simulink model "assignment3"  (R2016a)
settings: Solver=VariableStepAuto  StartTime=0.0  StopTime=1000  RelTol=1e-3
values from neighbouring files (symbols this model uses):
  f_ref = 0    [assgt3.m]
  Ki_f = 1/Ti_f    (= 0.215982721382)    [assgt3.m]
  Ki_p = 1/Ti_p    (= 0.289855072464)    [assgt3.m]
  Kp_f = 3.04    [assgt3.m]
  Kp_p = 18    [assgt3.m]
  p_ref = 0    [assgt3.m]
  Ti_f = 4.63    [assgt3.m]
  Ti_p = 3.45    [assgt3.m]
settings Model: Creator=Sondre  LastModifiedBy=Sondre

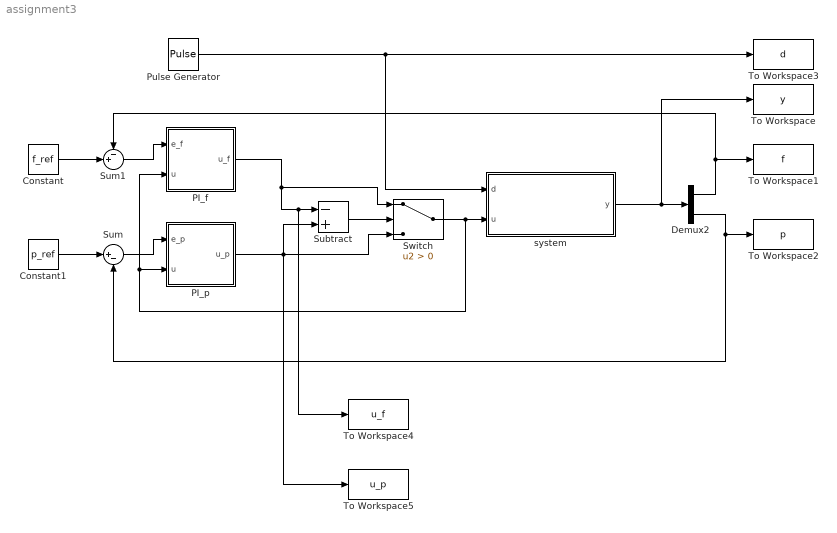
== system assignment3 ==
  Constant : Constant  Value=f_ref
  Constant1 : Constant  Value=p_ref
  Demux2 : Demux  Outputs=2
  PI_f : Subsystem
  PI_p : Subsystem
  Pulse Generator : DiscretePulseGenerator  PulseType=Time based  Period=500  PulseWidth=50
  Subtract : Sum  Inputs=-+
  Sum : Sum  Inputs=|+-
  Sum1 : Sum  Inputs=-+|
  Switch : Switch  Criteria=u2 > Threshold
  To Workspace : ToWorkspace  VariableName=y  SaveFormat=Timeseries  SampleTime=-1
  To Workspace1 : ToWorkspace  VariableName=f  SaveFormat=Timeseries  SampleTime=-1
  To Workspace2 : ToWorkspace  VariableName=p  SaveFormat=Timeseries  SampleTime=-1
  To Workspace3 : ToWorkspace  VariableName=d  SaveFormat=Timeseries  SampleTime=-1
  To Workspace4 : ToWorkspace  VariableName=u_f  SaveFormat=Timeseries  SampleTime=-1
  To Workspace5 : ToWorkspace  VariableName=u_p  SaveFormat=Timeseries  SampleTime=-1
  system : Subsystem
  wires:
  Demux2/2 -> Sum/2, To Workspace2/1
  system/1("y ") -> Demux2/1, To Workspace/1
  Constant1/1 -> Sum/1
  Sum/1 -> PI_p/1("e_p ")
  Sum1/1 -> PI_f/1("e_f ")
  PI_f/1("u_f ") -> Switch/1, To Workspace4/1, Subtract/1
  Pulse Generator/1 -> To Workspace3/1, system/1(d)
  Constant/1 -> Sum1/2
  Demux2/1 -> Sum1/1, To Workspace1/1
  PI_p/1("u_p ") -> To Workspace5/1, Subtract/2, Switch/3
  Subtract/1 -> Switch/2
  Switch/1 -> PI_f/2(u), PI_p/2("u "), system/2("u ")

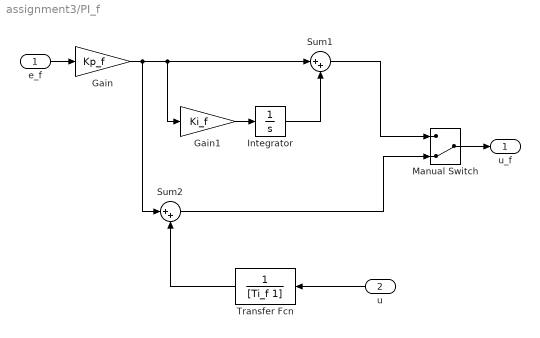
== system assignment3/PI_f ==
  "e_f " : Inport
  u : Inport  Port=2
  Gain : Gain  Gain=Kp_f
  Gain1 : Gain  Gain=Ki_f
  Integrator : Integrator
  Manual Switch : ManualSwitch  CurrentSetting=0
  Sum1 : Sum  Inputs=|++
  Sum2 : Sum  Inputs=|++
  Transfer Fcn : TransferFcn  Denominator=[Ti_f 1]
  "u_f " : Outport
  wires:
  Gain1/1 -> Integrator/1
  Integrator/1 -> Sum1/2
  "e_f "/1 -> Gain/1
  Gain/1 -> Sum2/1, Gain1/1, Sum1/1
  Sum2/1 -> Manual Switch/2
  Transfer Fcn/1 -> Sum2/2
  Manual Switch/1 -> "u_f "/1
  Sum1/1 -> Manual Switch/1
  u/1 -> Transfer Fcn/1

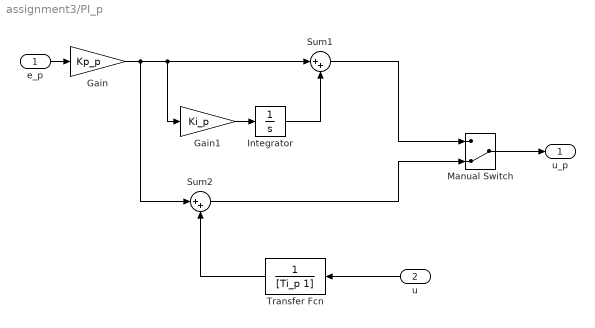
== system assignment3/PI_p ==
  "e_p " : Inport
  "u " : Inport  Port=2
  Gain : Gain  Gain=Kp_p
  Gain1 : Gain  Gain=Ki_p
  Integrator : Integrator
  Manual Switch : ManualSwitch  CurrentSetting=0
  Sum1 : Sum  Inputs=|++
  Sum2 : Sum  Inputs=|++
  Transfer Fcn : TransferFcn  Denominator=[Ti_p 1]
  "u_p " : Outport
  wires:
  Gain1/1 -> Integrator/1
  Integrator/1 -> Sum1/2
  "e_p "/1 -> Gain/1
  Gain/1 -> Sum2/1, Gain1/1, Sum1/1
  Sum2/1 -> Manual Switch/2
  Transfer Fcn/1 -> Sum2/2
  Manual Switch/1 -> "u_p "/1
  Sum1/1 -> Manual Switch/1
  "u "/1 -> Transfer Fcn/1

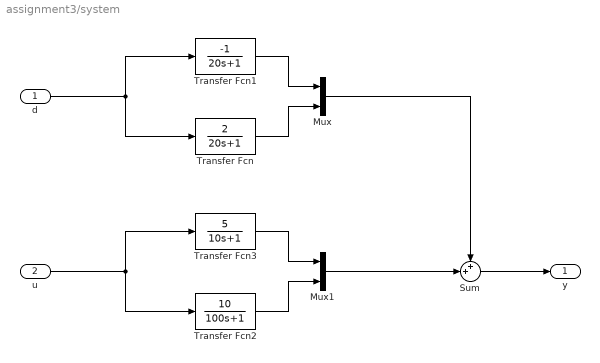
== system assignment3/system ==
  d : Inport
  "u " : Inport  Port=2
  Mux : Mux  Inputs=2
  Mux1 : Mux  Inputs=2
  Sum : Sum  Inputs=++|
  Transfer Fcn : TransferFcn  Numerator=[2]  Denominator=[20 1]
  Transfer Fcn1 : TransferFcn  Numerator=[-1]  Denominator=[20 1]
  Transfer Fcn2 : TransferFcn  Numerator=[10]  Denominator=[100 1]
  Transfer Fcn3 : TransferFcn  Numerator=[5]  Denominator=[10 1]
  "y " : Outport
  wires:
  "u "/1 -> Transfer Fcn2/1, Transfer Fcn3/1
  Transfer Fcn3/1 -> Mux1/1
  Transfer Fcn2/1 -> Mux1/2
  d/1 -> Transfer Fcn/1, Transfer Fcn1/1
  Sum/1 -> "y "/1
  Mux/1 -> Sum/1
  Transfer Fcn/1 -> Mux/2
  Mux1/1 -> Sum/2
  Transfer Fcn1/1 -> Mux/1
